simulink model "DynamicCompressionModel"  (R2019a)
settings: Solver=FixedStepDiscrete  StartTime=0.0  StopTime=t_end  RelTol=1e-3
InitFcn:
  | clear;
  | %DIAGNOSTIC = 0;  %% flag to give more information as simulation proceeds such as comments & plots
  | %CALIB_DIAGNOSTIC =  0; %% flag to give more information about calibration of filterbank due to overlap between filters: Mar 2016
  | %PRESCRIPT = 1;  %% flag to plot requested versus achieved insertion gains (esp for 125-250 Hz region).
  | %ipfiledigrms = -36; %% input file RMS in dB for 65 dB SPL equivalent
  | %opfiledigrms = -36; %% output file RMS in dB for 65 dB SPL equivalent
  | %equiv_ipSPL = 65; %% simulation of signal at this level through aid`
  | X_high = 1; % Maximum input
  | ref_dB = 85; X_ref = 1; % Define a reference point in X and its dBA value
  | % re_level = 10.^(.05*(equiv_ipSPL-65)); %% scale factor at start of hearing aid, to get input to desired simulation level
  | M_bits = 5;   % decides length of tables, 2^(4+M_bits)
  | 
  | NChans = 5;
  | [chan_cfs, ~ , t_atts, t_rels] ...
  |    = InitializeCompressionSettings(NChans);
  | % AidSettings5Chans;
  | 
  | %[VALID_WAV_FILE, sig, Fs, nbits, file_rms_dB, NStreams] ...
  | %  = loadwavfile(ipfiledigrms); %%  find [Fs], performs [recalculate] externally, provided valid file found
  | % VALID_WAV_FILE = 1;
  | [newfile, newpath] = uigetfile('*.wav','Open Signal File To Process.....');
  | if isequal(newfile,0) || isequal(newpath,0)
  |     fprintf(1,'\nFile not found'); VALID_WAV_FILE = 0;
  | else
  |     [sig, Fs] = audioread(strcat(newpath,newfile));
  | end
  | 
  | 
  | %% Test input: frequency sweep
  | X_thresh = 1*10^(0.05*(0-85));
  | Amplitudes = [X_thresh, X_thresh*10, X_thresh*100, X_thresh*1000, X_thresh*10000, 1]; %, X_thresh*100000];
  | 
  | %fMin = 100; %Hz
  | %fMax = 10000; %Hz
  | %Fs = 48000; %Hz
  | Fs_system = Fs;
  | Ts = 1/Fs;
  | Ts_system = Ts;
  | %tt = (0:length(sig)-1 )./Fs;
  | tt = 0:length(sig)-1;
  | tt = tt.*Ts;
  | %deltaF = (fMax - fMin)/tt(end);
  | %X_sweep = Amplitudes'*sin(2*pi*(fMin*tt +  0.5*deltaF*tt.*tt)) ;
  | 
  | %Volume = 6;
  | %sig = X_sweep(Volume,:)';
  | %% Replacing update_channel_params with only the needed pieces
  | 
  | % opplayer  = audioplayer(sig, Fs);
  | % nbits = opplayer.bitspersample;
  | %sig = resample(sig,48000,Fs);
  | %Fs = 48000;
  | 
  | 
  | % NStreams = min(size(sig));
  | EQ_SPAN_MSEC = 6;
  | 
  | insrt_frqs = [125, 250, 500, 1000, 2000, 3000, 4000, 6000, 8000, 10000 ]; %% decimal values
  | insrt_gns = [0 3 5 10 15 20 25 30 30 30]; %% prescribed dB for 65 dB input
  | %insrt_gns = 5*ones(1,length(insrt_frqs));  %no prescription
  | % n_insrts = length(insrt_gns);
  | 
  | UPPER_FREQ_LIM = min(11e3, 0.90*Fs/2);
  | 
  | % [ig_eq, calib_bpfs, dig_chan_lvl_0dBgain, dig_chan_dBthrs, Calib_recomb_dBpost] ...
  | %     = update_channel_params(Fs, NChans, chan_cfs, chan_thrs, insrt_frqs, insrt_gns, ...
  | %     0.1, UPPER_FREQ_LIM, EQ_SPAN_MSEC, PRESCRIPT, DIAGNOSTIC, CALIB_DIAGNOSTIC) ;  %% calculates channel edge frequencies, generates expected band levels for LTASS SWN to calibrate compressors & filterbank
  | [ig_eq, ~] = prescription_design_function(insrt_frqs, insrt_gns, Fs, EQ_SPAN_MSEC, 0); %% separate switch in [aid_sim] to turn off plotting.
  | %%% update_channel_params, to change edges array, as well as band levels when a channel cf changes.
  | edges = sqrt ( chan_cfs(2:end) .* chan_cfs(1:end-1) ); %% geometric mean
  | dummy_low_edge = edges(1)*(chan_cfs(1)/chan_cfs(2)); %% not used directly in Nchan_FbankAid, but helps with filter design, save for later
  | edges = [edges  UPPER_FREQ_LIM]; %% end stops to make software work, lowest not really implemented in software, upper set in main script
  | %%% spoof lowest edge freq for filyterbank design, not power calculations, does not produce edge in filterbank design
  | fb_edges = [dummy_low_edge  edges]; %% will need dummy low edge to make filterbank design software work, lowest not implemented in software other than transition width
  | [bpfs] = Nchan_FbankDesign(fb_edges, Fs, 0); %% Mar2016 move design of filterbank to here
  | 
  | calib_bpfs = bpfs; %% safety copy
  | % spec_size = 1024;
  | % bpzTotal= zeros(1,spec_size);
  | % bpCalzTotal = zeros(1,spec_size);
  | % Callibrate recombining gain? Or just fix bandpass FIRs to have unity peak gain.
  | % NOTE: Turns out bpfs have a pretty good peak unity gain. The combination
  | % of them all has a max error of -65 dBA (0.06%) above unity gain. That's fine.
  | %close(1); close(2);
  | % for(ix = 1:NChans)
  | %     [bpz(ix,:),bpFqs] = freqz(bpfs(2:(bpfs(1,ix)+1),ix),1,spec_size,Fs);
  | %     bpzMax(ix) = max(abs(bpz(ix,:)));
  | %     bpCalz(ix,:) = bpz(ix,:)./bpzMax(ix);
  | %     bpzTotal = bpzTotal + abs(bpz(ix,:));
  | %     bpCalzTotal = bpCalzTotal + abs(bpCalz(ix,:));
  | %     figure(1); hold on; semilogx(bpFqs, abs(bpz(ix,:)), 'b');
  | %     figure(2); hold on; semilogx(bpFqs, abs(bpCalz(ix,:)), 'g');
  | % end
  | % figure(1); hold on;
  | % semilogx(bpFqs, abs(bpzTotal), 'k'); %axis([100 12000 0 1.2]);
  | % xlabel('tested frqs(Hz)'); ylabel('Gain'); title('Original BP Response');
  | % figure(2); hold on;
  | % semilogx(bpFqs, abs(bpCalzTotal), 'k'); %axis([100 12000 0 1.2]);
  | % xlabel('tested frqs(Hz)'); ylabel('Gain'); title('Callibrated BP Response');
  | %%
  | 
  | % recombGain = 10.^(0.05.*Calib_recomb_dBpost);
  | recombGain = ones(1,NChans);
  | % translate sig into a form simulink likes
  | % Ts = 1/Fs;
  | % tt = (0:length(sig)-1).*Ts;
  | %t_end = tt(5*2^(M_bits+4) );   % to test table fill
  | t_end = tt(end);
  | sig_in = [tt', sig];
  | min_thresh_dB = 0;
  | for ix = 1:NChans
  |    [Gain_Table(:,ix), max_gain_prescript(ix), X_in(:,ix), chan_crs(ix)] ...
  |      = Compression_Wrapper_V2(Fs, min_thresh_dB, ...
  |      X_high, calib_bpfs(:,ix), ig_eq, ref_dB, X_ref, M_bits);
  | end
  | 
  | Initialize_Delay_Values;
  | %chan_recomb_gain = 10.^((0.05*Calib_recomb_dBpost));
  | W_bits = 32;
  | F_bits = 28;
  | M_bits = 5;
  | M_Bits = M_bits;
  | 
  | % Generating signals for simulink
  | Table_Fill = zeros(1,length(tt))';
  | %Table_Fill(1) = Gain_Table(end,5);
  | Table_Fill(1                : 2^(M_bits+4) )  = Gain_Table(:,1);
  | Table_Fill(2^(M_bits+4)+1   : 2*2^(M_bits+4) )= Gain_Table(:,2);
  | Table_Fill(2*2^(M_bits+4)+1 : 3*2^(M_bits+4) )= Gain_Table(:,3);
  | Table_Fill(3*2^(M_bits+4)+1 : 4*2^(M_bits+4) )= Gain_Table(:,4);
  | Table_Fill(4*2^(M_bits+4)+1 : 5*2^(M_bits+4) )= Gain_Table(:,5);
  | Table_Fill_t = [tt', zeros(1,length(tt))'];
  | Fill_Valid = zeros(1,length(tt))';
  | % Fill_Valid(1:5*2^(M_bits+4)) = 1;
  | % Fill_Valid = boolean(Fill_Valid);
  | Fill_Valid_t = [tt', Fill_Valid];
  | t_att = t_atts./1000; s_att = t_att.*Fs; % change units of t_atts from ms to samples
  | t_rel = t_rels./1000; s_rel = t_rel.*Fs; % change units of t_rels from ms to samples
  | r_att = nthroot(0.1, s_att);
  | r_rel = nthroot(0.1, s_rel);
  | 
  | Reset = [tt', boolean(zeros(1,length(tt)))'];
StopFcn:
  | proc_sig = double(out.proc_sig.data(:));
  | %alignedSigs = double(out.alignedSigs.data(:));
  | %[opwav, stop_ok] = savewavfile(opfiledigrms, ipfiledigrms, proc_sig, Fs, nbits, NStreams);
  | 
  | %load('SweepSimOutput.mat')
  | %X_out_Sweep_Sim(Volume,:) = proc_sig;
  | %save('SweepSimOutput.mat', 'X_out_Sweep_Sim');
values from neighbouring files (symbols this model uses):
  chan_cfs = [125 185 255 337 433 545 676 829 1008 1216 1460 1746 2079 2468 2923 3455 4077 4804 5653 6645 7805 9161]    [AidSettings22Chans.m]    (also in AidSettings3Chans.m = [750 1500 4000 ]; AidSettings5Chans.m = [500 1000 2000 4000 8000]; AidSettingsXChans.m = a*r.^(1:NChans); InitializeCompressionSettings.m = a*r.^(1:NChans))
  delayFix = maxDelay-delays    [Initialize_Delay_Values.m]    (also in cCompileTest.m = zeros(1,5))
  Fs = 48000    [cCompileTest.m]    (also in errorTesting.m; fft_compute_ASDF.m = 16000; fixedPointTesting.m; plotting_stuff.m)
  ig_eq = zeros(1,289)    [cCompileTest.m]
  sig = sig * 10.^(.05*adjustdB)    [loadwavfile.m]    (also in testing.m = X_sweep(Volume,:)')
  t_atts = [10 10 10 10 10 10 10 10 10 10 10 10 10 10 10 10 10 10 10 10 10 10]    [AidSettings22Chans.m]    (also in AidSettings3Chans.m = [200 100 100]; AidSettings5Chans.m = [200 100 100 100 100]; InitializeCompressionSettings.m = zeros(1,5))
  t_rels = [100 100 100 100 100 100 100 100 100 100 100 100 100 100 100 100 100 100 100 100 100 100]    [AidSettings22Chans.m]    (also in AidSettings3Chans.m = [2000 1500 1200 ]; AidSettings5Chans.m = [2000 1500 1200 1000 1000]; InitializeCompressionSettings.m = zeros(1,5))
libraries: simulink x352, hdlsllib x258, dsphdlfiltering x1
(part 1 of 7)
settings Model: DataTypeOverride=Off  Creator=Bailey  LastModifiedBy=Bailey
settings DataIOCC: InitialState=Table_Fill(1: 2^(M_bits+4) )  SaveOutput=off  SaveTime=off
settings OptimizationCC: BlockReduction=off  ConditionallyExecuteInputs=off  DefaultParameterBehavior=Inlined
settings DebuggingCC: AlgebraicLoopMsg=error  SingleTaskRateTransMsg=error
settings HardwareCC: ProdBitPerPointer=32  ProdBitPerSizeT=32  ProdBitPerPtrDiffT=32  ProdLargestAtomicFloat=None  ProdIntDivRoundTo=Undefined  ProdEndianess=Unspecified  ProdWordSize=32  ProdHWDeviceType=ASIC/FPGA->ASIC/FPGA  TargetBitPerPointer=64  TargetBitPerSizeT=64  TargetBitPerPtrDiffT=64  TargetLongLongMode=on  TargetIntDivRoundTo=Zero  TargetEndianess=LittleEndian  TargetWordSize=64  TargetHWDeviceType=Custom Processor->MATLAB Host Computer  ProdEqTarget=off

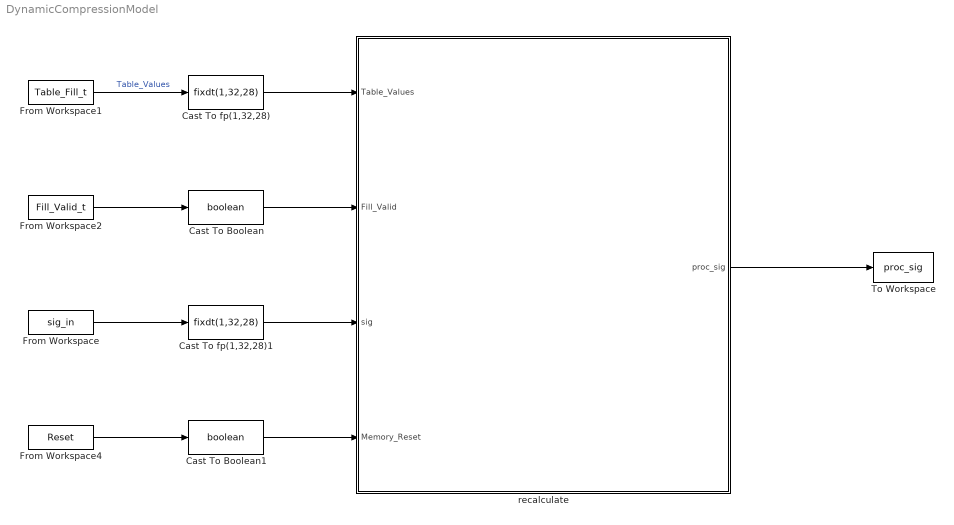
== system DynamicCompressionModel ==
  Cast To Boolean : DataTypeConversion  OutDataTypeStr=boolean
  Cast To Boolean1 : DataTypeConversion  OutDataTypeStr=boolean
  Cast To fp(1,32,28) : DataTypeConversion  OutDataTypeStr=fixdt(1,32,28)  RndMeth=Round
  Cast To fp(1,32,28)1 : DataTypeConversion  OutDataTypeStr=fixdt(1,32,28)  RndMeth=Round
  From Workspace : FromWorkspace  VariableName=sig_in  SampleTime=Ts  OutputAfterFinalValue=Setting to zero
  From Workspace1 : FromWorkspace  VariableName=Table_Fill_t  SampleTime=Ts  Interpolate=off  OutputAfterFinalValue=Setting to zero
  From Workspace2 : FromWorkspace  VariableName=Fill_Valid_t  SampleTime=Ts  OutputAfterFinalValue=Setting to zero
  From Workspace4 : FromWorkspace  VariableName=Reset  SampleTime=Ts  Interpolate=off  OutputAfterFinalValue=Setting to zero
  To Workspace : ToWorkspace  VariableName=proc_sig  SaveFormat=Timeseries  SampleTime=-1
  recalculate : Subsystem
  wires:
  From Workspace/1 -> Cast To fp(1,32,28)1/1
  recalculate/1(proc_sig) -> To Workspace/1
  From Workspace1/1 -> Cast To fp(1,32,28)/1  "Table_Values"
  From Workspace4/1 -> Cast To Boolean1/1
  Cast To Boolean/1 -> recalculate/2(Fill_Valid)
  From Workspace2/1 -> Cast To Boolean/1
  Cast To Boolean1/1 -> recalculate/4(Memory_Reset)
  Cast To fp(1,32,28)/1 -> recalculate/1(Table_Values)
  Cast To fp(1,32,28)1/1 -> recalculate/3(sig)

== system DynamicCompressionModel/recalculate ==
  note: High Clipping
  note: Prescription Application
  note: Low Clipping
  Table_Values : Inport
  Fill_Valid : Inport  Port=2
  sig : Inport  Port=3
  Memory_Reset : Inport  Port=4
  Compare To Constant : simulink/Logic and Bit Operations/Compare To Constant  relop=>=  const=X_high  OutDataTypeStr=boolean
  Compare To Constant1 : simulink/Logic and Bit Operations/Compare To Constant  relop=<=  const=-X_high  OutDataTypeStr=boolean
  Constant : Constant  Value=X_high  OutDataTypeStr=fixdt(1,W_bits, F_bits)  SampleTime=-1
  Constant1 : Constant  Value=-X_high  OutDataTypeStr=fixdt(1,W_bits, F_bits)  SampleTime=-1
  Nchan_FbankAGC_AID : Subsystem
  Switch : Switch  Criteria=u2 ~= 0
  Switch1 : Switch  Criteria=u2 ~= 0
  ig65 fir : DiscreteFir  Coefficients=ig_eq  CoefDataTypeStr=fixdt(1, W_bits*2, W_bits)  ProductDataTypeStr=fixdt(1, W_bits*2, W_bits)  AccumDataTypeStr=fixdt(1, W_bits*2, W_bits)  OutDataTypeStr=fixdt(1, W_bits, F_bits)
  proc_sig : Outport
  wires:
  sig/1 -> Nchan_FbankAGC_AID/3(input_signal)
  Table_Values/1 -> Nchan_FbankAGC_AID/1(Table_Values)
  Fill_Valid/1 -> Nchan_FbankAGC_AID/2(Fill_Valid)
  Memory_Reset/1 -> Nchan_FbankAGC_AID/4(Reset)
  ig65 fir/1 -> Compare To Constant/1, Switch/3  "re_level.*eq_sig"
  Nchan_FbankAGC_AID/1(proc_sig) -> ig65 fir/1
  Compare To Constant/1 -> Switch/2
  Constant/1 -> Switch/1
  Switch/1 -> Switch1/3, Compare To Constant1/1
  Compare To Constant1/1 -> Switch1/2
  Constant1/1 -> Switch1/1
  Switch1/1 -> proc_sig/1

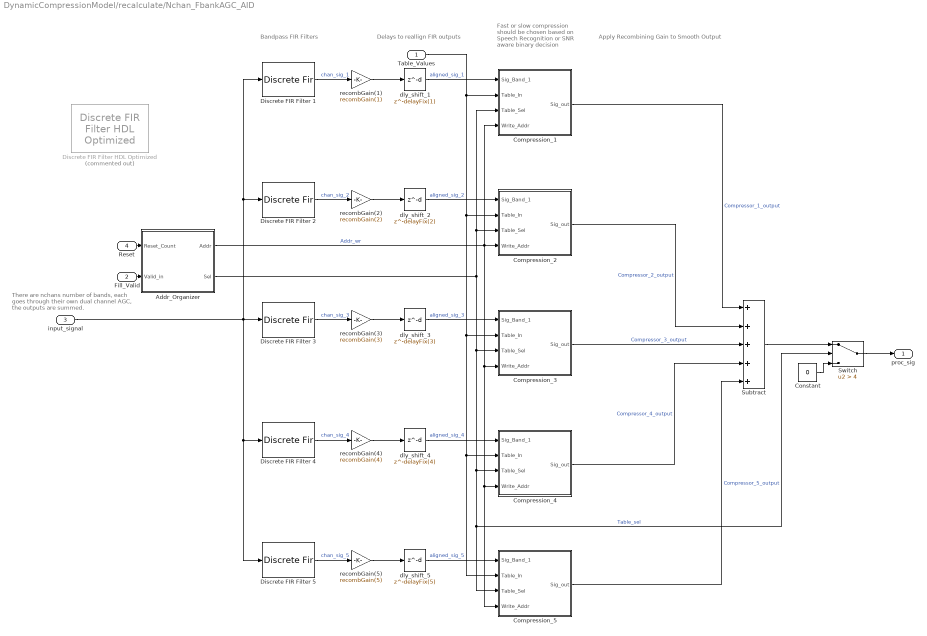
== system DynamicCompressionModel/recalculate/Nchan_FbankAGC_AID ==
  note: Apply Recombining Gain to Smooth Output
  note: Fast or slow compression
      | should be chosen based
      | on Speech Recognition or
      | SNR aware binary decision
  note: Delays to reallign FIR outputs
  note: Bandpass FIR Filters
  note: There are nchans number of bands,
      |  each goes through their own dual
      | channel AGC, the outputs are summed.
  Table_Values : Inport
  Fill_Valid : Inport  Port=2
  input_signal : Inport  Port=3
  Reset : Inport  Port=4
  Addr_Organizer : Subsystem
  Compression_1 : Subsystem
  Compression_2 : Subsystem
  Compression_3 : Subsystem
  Compression_4 : Subsystem
  Compression_5 : Subsystem
  Constant : Constant  Value=0  OutDataTypeStr=fixdt(1,W_bits, F_bits)  SampleTime=-1
  Discrete FIR Filter HDL Optimized : dsphdlfiltering/Discrete FIR Filter HDL Optimized  Commented=on  NumeratorSource=Property  Numerator=[ 0.5, 0.5 ]  NumeratorPrototype=[ 0.5, 0.5 ]  FilterStructure=Direct form systolic  SerializationOption=Minimum number of cycles between valid input samples  NumberOfCycles=2  NumberOfMultipliers=2  SimulateUsing=Code generation  roundingMode=Floor  overflowMode=off  CoefficientsDataTypeStr=Inherit: Same word length as input  CoefficientsMin=[]  CoefficientsMax=[]  OutputMin=[]  OutputMax=[]  ResetInputPort=off  HDLGlobalReset=off
      settings: SourceProductName=DSP System Toolbox  SourceProductBaseCode=DS
  Discrete FIR Filter 1 : DiscreteFir  Coefficients=calib_bpfs(2:calib_bpfs(1,1)+1 ,1)'  SampleTime=Ts  CoefDataTypeStr=fixdt(1, W_bits, F_bits)  ProductDataTypeStr=fixdt(1, W_bits, F_bits)  AccumDataTypeStr=fixdt(1, W_bits, F_bits)  OutDataTypeStr=fixdt(1, W_bits, F_bits)
  Discrete FIR Filter 2 : DiscreteFir  Coefficients=calib_bpfs(2:calib_bpfs(1,2)+1 ,2)'  CoefDataTypeStr=fixdt(1, W_bits, F_bits)  ProductDataTypeStr=fixdt(1, W_bits, F_bits)  AccumDataTypeStr=fixdt(1, W_bits, F_bits)  OutDataTypeStr=fixdt(1, W_bits, F_bits)
  Discrete FIR Filter 3 : DiscreteFir  Coefficients=calib_bpfs(2:calib_bpfs(1,3)+1 ,3)'  CoefDataTypeStr=fixdt(1, W_bits, F_bits)  ProductDataTypeStr=fixdt(1, W_bits, F_bits)  AccumDataTypeStr=fixdt(1, W_bits, F_bits)  OutDataTypeStr=fixdt(1, W_bits, F_bits)
  Discrete FIR Filter 4 : DiscreteFir  Coefficients=calib_bpfs(2:calib_bpfs(1,4)+1 ,4)'  CoefDataTypeStr=fixdt(1, W_bits, F_bits)  ProductDataTypeStr=fixdt(1, W_bits, F_bits)  AccumDataTypeStr=fixdt(1, W_bits, F_bits)  OutDataTypeStr=fixdt(1, W_bits, F_bits)
  Discrete FIR Filter 5 : DiscreteFir  Coefficients=calib_bpfs(2:calib_bpfs(1,5)+1 ,5)'  CoefDataTypeStr=fixdt(1, W_bits, F_bits)  ProductDataTypeStr=fixdt(1, W_bits, F_bits)  AccumDataTypeStr=fixdt(1, W_bits, F_bits)  OutDataTypeStr=fixdt(1, W_bits, F_bits)
  Subtract : Sum  Inputs=+++++
  Switch : Switch  Criteria=u2 > Threshold  Threshold=4
  dly_shift_1 : Delay  DelayLength=delayFix(1)  DelayLengthUpperLimit=500
  dly_shift_2 : Delay  DelayLength=delayFix(2)  DelayLengthUpperLimit=500
  dly_shift_3 : Delay  DelayLength=delayFix(3)  DelayLengthUpperLimit=500
  dly_shift_4 : Delay  DelayLength=delayFix(4)  DelayLengthUpperLimit=500
  dly_shift_5 : Delay  DelayLength=delayFix(5)  DelayLengthUpperLimit=500
  recombGain(1) : Gain  Gain=recombGain(1)  OutDataTypeStr=Inherit: Same as input
  recombGain(2) : Gain  Gain=recombGain(2)  OutDataTypeStr=Inherit: Same as input
  recombGain(3) : Gain  Gain=recombGain(3)  OutDataTypeStr=Inherit: Same as input
  recombGain(4) : Gain  Gain=recombGain(4)  OutDataTypeStr=Inherit: Same as input
  recombGain(5) : Gain  Gain=recombGain(5)  OutDataTypeStr=Inherit: Same as input
  proc_sig : Outport
  wires:
  Discrete FIR Filter 1/1 -> recombGain(1)/1  "chan_sig_1"
  dly_shift_1/1 -> Compression_1/1(Sig_Band_1)  "aligned_sig_1"
  Compression_1/1(Sig_out) -> Subtract/1  "Compressor_1_output"
  dly_shift_2/1 -> Compression_2/1(Sig_Band_1)  "aligned_sig_2"
  Discrete FIR Filter 2/1 -> recombGain(2)/1  "chan_sig_2"
  dly_shift_3/1 -> Compression_3/1(Sig_Band_1)  "aligned_sig_3"
  Discrete FIR Filter 3/1 -> recombGain(3)/1  "chan_sig_3"
  Discrete FIR Filter 5/1 -> recombGain(5)/1  "chan_sig_5"
  input_signal/1 -> Discrete FIR Filter 5/1, Discrete FIR Filter 4/1, Discrete FIR Filter 2/1, Discrete FIR Filter 1/1, Discrete FIR Filter 3/1
  dly_shift_5/1 -> Compression_5/1(Sig_Band_1)  "aligned_sig_5"
  dly_shift_4/1 -> Compression_4/1(Sig_Band_1)  "aligned_sig_4"
  Discrete FIR Filter 4/1 -> recombGain(4)/1  "chan_sig_4"
  Compression_3/1(Sig_out) -> Subtract/3  "Compressor_3_output"
  Compression_2/1(Sig_out) -> Subtract/2  "Compressor_2_output"
  Compression_4/1(Sig_out) -> Subtract/4  "Compressor_4_output"
  Compression_5/1(Sig_out) -> Subtract/5  "Compressor_5_output"
  Addr_Organizer/1(Addr) -> Compression_3/4(Write_Addr), Compression_5/4(Write_Addr), Compression_4/4(Write_Addr), Compression_2/4(Write_Addr), Compression_1/4(Write_Addr)  "Addr_wr"
  Reset/1 -> Addr_Organizer/1(Reset_Count)
  Fill_Valid/1 -> Addr_Organizer/2(Valid_in)
  Table_Values/1 -> Compression_5/2(Table_In), Compression_4/2(Table_In), Compression_3/2(Table_In), Compression_2/2(Table_In), Compression_1/2(Table_In)
  Addr_Organizer/2(Sel) -> Compression_3/3(Table_Sel), Compression_5/3(Table_Sel), Switch/2, Compression_4/3(Table_Sel), Compression_1/3(Table_Sel), Compression_2/3(Table_Sel)  "Table_sel"
  Subtract/1 -> Switch/1
  Constant/1 -> Switch/3
  Switch/1 -> proc_sig/1
  recombGain(1)/1 -> dly_shift_1/1
  recombGain(2)/1 -> dly_shift_2/1
  recombGain(3)/1 -> dly_shift_3/1
  recombGain(4)/1 -> dly_shift_4/1
  recombGain(5)/1 -> dly_shift_5/1

== system DynamicCompressionModel/recalculate/Nchan_FbankAGC_AID/Addr_Organizer ==
  note: Addr line contains the local address bits: 0-63
  note: Select Line is 000 to 101, if 110 writing is complete
  Reset_Count : Inport
  Valid_in : Inport  Port=2
  Bit Slice : hdlsllib/Logic and Bit Operations/Bit Slice  lidx=3+M_bits  ridx=0
      settings: SourceProductName=Simulink  SourceProductBaseCode=SL
  Bit Slice1 : hdlsllib/Logic and Bit Operations/Bit Slice  lidx=6+M_bits  ridx=4+M_bits
      settings: SourceProductName=Simulink  SourceProductBaseCode=SL
  Counter_up_to_320 : hdlsllib/Sources/HDL Counter  CountType=Count limited  CountInit=5*2^(4+M_Bits)  CountStep=1  CountMax=5*2^(4+M_Bits)+1  CountFromType=Initial value  CountFrom=5*2^(4+M_Bits)  CountResetPort=on  CountLoadPort=off  CountEnbPort=on  CountDirPort=off  CountDataType=Unsigned  CountWordLen=7+M_Bits  CountFracLen=0  CountSampTime=1
      settings: SourceProductName=Simulink
  Data Type Conversion : DataTypeConversion  OutDataTypeStr=fixdt(0,7+M_Bits,0)
  Data Type Conversion1 : DataTypeConversion  OutDataTypeStr=fixdt(0,4+M_bits,0)
  Data Type Conversion2 : DataTypeConversion  OutDataTypeStr=fixdt(0,3,0)
  Addr : Outport
  Sel : Outport  Port=2
  wires:
  Valid_in/1 -> Counter_up_to_320/2
  Reset_Count/1 -> Counter_up_to_320/1
  Counter_up_to_320/1 -> Data Type Conversion/1
  Data Type Conversion/1 -> Bit Slice1/1, Bit Slice/1
  Bit Slice1/1 -> Data Type Conversion2/1  "top3Bits"
  Bit Slice/1 -> Data Type Conversion1/1
  Data Type Conversion1/1 -> Addr/1
  Data Type Conversion2/1 -> Sel/1

== system DynamicCompressionModel/recalculate/Nchan_FbankAGC_AID/Compression_1 ==
  note: Calculate Compression Gain Needed
  note: Apply to the Envelope
  Sig_Band_1 : Inport
  Table_In : Inport  Port=2
  Table_Sel : Inport  Port=3
  Write_Addr : Inport  Port=4
  Compare To Constant : simulink/Logic and Bit Operations/Compare To Constant  relop===  const=0  OutDataTypeStr=boolean
  Compression_Envelope : Subsystem
  Compression_Gain_Calc : Subsystem
  Constant : Constant  Value=0  OutDataTypeStr=fixdt(1,W_bits,F_bits)  SampleTime=-1
  Data Type Conversion1 : DataTypeConversion  OutDataTypeStr=fixdt(1,W_bits,F_bits)
  Delay : Delay  DelayLength=3
  Product : Product
  Switch : Switch  Criteria=u2 > Threshold  Threshold=4  ZeroCross=off
  Unit Delay : UnitDelay  InitialCondition=1  SampleTime=-1  HasFrameUpgradeWarning=on
  Sig_out : Outport
  wires:
  Compression_Envelope/1(Gain_Out) -> Product/1, Unit Delay/1
  Unit Delay/1 -> Compression_Envelope/2(Curr_Gain)
  Product/1 -> Data Type Conversion1/1
  Compare To Constant/1 -> Compression_Gain_Calc/3(Table_Fill_Valid)
  Write_Addr/1 -> Compression_Gain_Calc/2(Write_Addr)
  Table_In/1 -> Compression_Gain_Calc/1(Table_Fill)  "Table_Values"
  Switch/1 -> Delay/1
  Table_Sel/1 -> Compare To Constant/1, Switch/2
  Constant/1 -> Switch/3
  Sig_Band_1/1 -> Compression_Gain_Calc/4(Data_In), Switch/1
  Data Type Conversion1/1 -> Sig_out/1
  Delay/1 -> Product/2
  Compression_Gain_Calc/1(Gain_C_out) -> Compression_Envelope/1(Desired_Gain)

== system DynamicCompressionModel/recalculate/Nchan_FbankAGC_AID/Compression_2 ==
  note: Calculate Compression Gain Needed
  note: Apply to the Envelope
  Sig_Band_1 : Inport
  Table_In : Inport  Port=2
  Table_Sel : Inport  Port=3
  Write_Addr : Inport  Port=4
  Compare To Constant : simulink/Logic and Bit Operations/Compare To Constant  relop===  const=1  OutDataTypeStr=boolean
  Compression_Envelope : Subsystem
  Compression_Gain_Calc : Subsystem
  Constant : Constant  Value=0  OutDataTypeStr=fixdt(1,W_bits,F_bits)  SampleTime=-1
  Data Type Conversion1 : DataTypeConversion  OutDataTypeStr=fixdt(1,W_bits,F_bits)
  Delay : Delay  DelayLength=3
  Product : Product
  Switch : Switch  Criteria=u2 > Threshold  Threshold=4  ZeroCross=off
  Unit Delay : UnitDelay  InitialCondition=1  SampleTime=-1  HasFrameUpgradeWarning=on
  Sig_out : Outport
  wires:
  Compression_Envelope/1(Gain_Out) -> Product/1, Unit Delay/1
  Unit Delay/1 -> Compression_Envelope/2(Curr_Gain)
  Compare To Constant/1 -> Compression_Gain_Calc/3(Table_Fill_Valid)
  Write_Addr/1 -> Compression_Gain_Calc/2(Write_Addr)
  Table_In/1 -> Compression_Gain_Calc/1(Table_Fill)  "Table_Values"
  Table_Sel/1 -> Compare To Constant/1, Switch/2
  Constant/1 -> Switch/3
  Switch/1 -> Delay/1
  Sig_Band_1/1 -> Compression_Gain_Calc/4(Data_In), Switch/1
  Product/1 -> Data Type Conversion1/1
  Data Type Conversion1/1 -> Sig_out/1
  Delay/1 -> Product/2
  Compression_Gain_Calc/1(Gain_C_out) -> Compression_Envelope/1(Desired_Gain)

== system DynamicCompressionModel/recalculate/Nchan_FbankAGC_AID/Compression_3 ==
  note: Calculate Compression Gain Needed
  note: Apply to the Envelope
  Sig_Band_1 : Inport
  Table_In : Inport  Port=2
  Table_Sel : Inport  Port=3
  Write_Addr : Inport  Port=4
  Compare To Constant : simulink/Logic and Bit Operations/Compare To Constant  relop===  const=2  OutDataTypeStr=boolean
  Compression_Envelope : Subsystem
  Compression_Gain_Calc : Subsystem
  Constant : Constant  Value=0  OutDataTypeStr=fixdt(1,W_bits,F_bits)  SampleTime=-1
  Data Type Conversion1 : DataTypeConversion  OutDataTypeStr=fixdt(1,W_bits,F_bits)
  Delay : Delay  DelayLength=3
  Product : Product
  Switch : Switch  Criteria=u2 > Threshold  Threshold=4  ZeroCross=off
  Unit Delay : UnitDelay  InitialCondition=1  SampleTime=-1  HasFrameUpgradeWarning=on
  Sig_out : Outport
  wires:
  Compression_Envelope/1(Gain_Out) -> Product/1, Unit Delay/1
  Unit Delay/1 -> Compression_Envelope/2(Curr_Gain)
  Compare To Constant/1 -> Compression_Gain_Calc/3(Table_Fill_Valid)
  Write_Addr/1 -> Compression_Gain_Calc/2(Write_Addr)
  Table_In/1 -> Compression_Gain_Calc/1(Table_Fill)  "Table_Values"
  Switch/1 -> Delay/1
  Table_Sel/1 -> Compare To Constant/1, Switch/2
  Constant/1 -> Switch/3
  Sig_Band_1/1 -> Compression_Gain_Calc/4(Data_In), Switch/1
  Product/1 -> Data Type Conversion1/1
  Data Type Conversion1/1 -> Sig_out/1
  Delay/1 -> Product/2
  Compression_Gain_Calc/1(Gain_C_out) -> Compression_Envelope/1(Desired_Gain)

== system DynamicCompressionModel/recalculate/Nchan_FbankAGC_AID/Compression_4 ==
  note: Calculate Compression Gain Needed
  note: Apply to the Envelope
  Sig_Band_1 : Inport
  Table_In : Inport  Port=2
  Table_Sel : Inport  Port=3
  Write_Addr : Inport  Port=4
  Compare To Constant : simulink/Logic and Bit Operations/Compare To Constant  relop===  const=3  OutDataTypeStr=boolean
  Compression_Envelope : Subsystem
  Compression_Gain_Calc : Subsystem
  Constant : Constant  Value=0  OutDataTypeStr=fixdt(1,W_bits,F_bits)  SampleTime=-1
  Data Type Conversion1 : DataTypeConversion  OutDataTypeStr=fixdt(1,W_bits,F_bits)
  Delay : Delay  DelayLength=3
  Product : Product
  Switch : Switch  Criteria=u2 > Threshold  Threshold=4  ZeroCross=off
  Unit Delay : UnitDelay  InitialCondition=1  SampleTime=-1  HasFrameUpgradeWarning=on
  Sig_out : Outport
  wires:
  Compression_Envelope/1(Gain_Out) -> Product/1, Unit Delay/1
  Unit Delay/1 -> Compression_Envelope/2(Curr_Gain)
  Compare To Constant/1 -> Compression_Gain_Calc/3(Table_Fill_Valid)
  Compression_Gain_Calc/1(Gain_C_out) -> Compression_Envelope/1(Desired_Gain)
  Write_Addr/1 -> Compression_Gain_Calc/2(Write_Addr)
  Table_In/1 -> Compression_Gain_Calc/1(Table_Fill)  "Table_Values"
  Switch/1 -> Delay/1
  Table_Sel/1 -> Compare To Constant/1, Switch/2
  Constant/1 -> Switch/3
  Sig_Band_1/1 -> Compression_Gain_Calc/4(Data_In), Switch/1
  Product/1 -> Data Type Conversion1/1
  Data Type Conversion1/1 -> Sig_out/1
  Delay/1 -> Product/2

== system DynamicCompressionModel/recalculate/Nchan_FbankAGC_AID/Compression_5 ==
  note: Calculate Compression Gain Needed
  note: Apply to the Envelope
  Sig_Band_1 : Inport
  Table_In : Inport  Port=2
  Table_Sel : Inport  Port=3
  Write_Addr : Inport  Port=4
  Compare To Constant : simulink/Logic and Bit Operations/Compare To Constant  relop===  const=4  OutDataTypeStr=boolean
  Compression_Envelope : Subsystem
  Compression_Gain_Calc : Subsystem
  Constant : Constant  Value=0  OutDataTypeStr=fixdt(1,W_bits,F_bits)  SampleTime=-1
  Data Type Conversion1 : DataTypeConversion  OutDataTypeStr=fixdt(1,W_bits,F_bits)
  Delay : Delay  DelayLength=3
  Product : Product
  Switch : Switch  Criteria=u2 > Threshold  Threshold=4  ZeroCross=off
  Unit Delay : UnitDelay  InitialCondition=1  SampleTime=-1  HasFrameUpgradeWarning=on
  Sig_out : Outport
  wires:
  Compression_Envelope/1(Gain_Out) -> Product/1, Unit Delay/1
  Unit Delay/1 -> Compression_Envelope/2(Curr_Gain)
  Compare To Constant/1 -> Compression_Gain_Calc/3(Table_Fill_Valid)
  Compression_Gain_Calc/1(Gain_C_out) -> Compression_Envelope/1(Desired_Gain)
  Write_Addr/1 -> Compression_Gain_Calc/2(Write_Addr)
  Table_In/1 -> Compression_Gain_Calc/1(Table_Fill)  "Table_Values"
  Switch/1 -> Delay/1
  Table_Sel/1 -> Compare To Constant/1, Switch/2
  Constant/1 -> Switch/3
  Sig_Band_1/1 -> Compression_Gain_Calc/4(Data_In), Switch/1
  Product/1 -> Data Type Conversion1/1
  Data Type Conversion1/1 -> Sig_out/1
  Delay/1 -> Product/2

== system DynamicCompressionModel/recalculate/Nchan_FbankAGC_AID/Compression_1/Compression_Envelope ==
  note: Curr > Desired:
      | Attack
  note: Curr < Desired:
      | Release
  Desired_Gain : Inport
  Curr_Gain : Inport  Port=2
  Attack_Envelope : Subsystem  TreatAsAtomicUnit=on
  Compare To Zero : simulink/Logic and Bit Operations/Compare To Zero  relop=>=  OutDataTypeStr=boolean
  Logical Operator : Logic  Operator=NOT  AllPortsSameDT=off  OutDataTypeStr=boolean
  Release_Envelope : Subsystem  TreatAsAtomicUnit=on
  Subtract : Sum  Inputs=-+  AccumDataTypeStr=fixdt(1,W_bits,F_bits)  OutDataTypeStr=Inherit: Same as accumulator
  Switch : Switch
  Gain_Out : Outport
  wires:
  Desired_Gain/1 -> Attack_Envelope/2(Desired), Release_Envelope/2(Desired), Subtract/1
  Curr_Gain/1 -> Attack_Envelope/1(Curr), Subtract/2, Release_Envelope/1(Curr)
  Subtract/1 -> Switch/2, Compare To Zero/1
  Compare To Zero/1 -> Attack_Envelope/Enable, Logical Operator/1
  Logical Operator/1 -> Release_Envelope/Enable
  Switch/1 -> Gain_Out/1
  Attack_Envelope/1(Gain_out) -> Switch/1
  Release_Envelope/1(Gain_out) -> Switch/3

== system DynamicCompressionModel/recalculate/Nchan_FbankAGC_AID/Compression_1/Compression_Gain_Calc ==
  note: Data_In assumed before applied prescription FIR
  note: Compression: Assume the input is a single band coming from the system.
      |
      | Goals:
      | 	- Take in a single point
      | 	- compare the volume to a known hard cap for the data
      | 	- attenuate the signal if it's above a certain threshold
      | 		- the distance above the threshold should be cut in dB by a ratio R
      | 	- return the output point at the same sample rate received
  Table_Fill : Inport
  Write_Addr : Inport  Port=2
  Table_Fill_Valid : Inport  Port=3
  Data_In : Inport  Port=4
  Abs : Abs
  Constant : Constant  OutDataTypeStr=fixdt(0,9,0)  SampleTime=-1
  High_Gain_Table : Subsystem  AncestorBlock=hdlsllibUNLOCKED/HDL RAMs/Dual Port RAM  mask(Dual-port RAM){ram_size=4+M_Bits}
      mask prompts: ram_size "Address port width (2 to 29 bits)"
      mask help: This block simulates a dual-port RAM with two data output ports.
      mask init:
      | hdlblkmask_dpram;
      mask Help: helpview([docroot '/simulink/helptargets.map'],'HDL_dual_port_RAM');
  Linear_Approximation : Subsystem
  LogAddressing : Subsystem
  Low_Gain_Table : Subsystem  mask(Dual-port RAM){ram_size=4+M_Bits}
      mask prompts: ram_size "Address port width (2 to 29 bits)"
      mask help: This block simulates a dual-port RAM with two data output ports.
      mask init:
      | hdlblkmask_dpram;
      mask Help: helpview([docroot '/simulink/helptargets.map'],'HDL_dual_port_RAM');
  Subtract : Sum  OutDataTypeStr=Inherit: Same as first input
  Terminator : Terminator
  Terminator1 : Terminator
  Unit Delay1 : UnitDelay  InitialCondition=1  SampleTime=-1  HasFrameUpgradeWarning=on
  Unit Delay2 : UnitDelay  InitialCondition=1  SampleTime=-1  HasFrameUpgradeWarning=on
  Unit Delay3 : UnitDelay  InitialCondition=1  SampleTime=-1  HasFrameUpgradeWarning=on
  Gain_C_out : Outport
  wires:
  Table_Fill/1 -> High_Gain_Table/1(wr_din), Low_Gain_Table/1(wr_din)
  Table_Fill_Valid/1 -> High_Gain_Table/3(wr_en), Low_Gain_Table/3(wr_en)
  Write_Addr/1 -> High_Gain_Table/2(wr_addr), Low_Gain_Table/2(wr_addr)
  LogAddressing/1(addr_r) -> Low_Gain_Table/4(rd_addr), Unit Delay3/1, Subtract/1  "addr_low"
  Abs/1 -> Unit Delay2/1, LogAddressing/1(x_in)  "|X_in|"
  Data_In/1 -> Abs/1
  Constant/1 -> Subtract/2
  Subtract/1 -> High_Gain_Table/4(rd_addr)  "addr_high"
  Low_Gain_Table/1(wr_dout) -> Terminator/1
  High_Gain_Table/1(wr_dout) -> Terminator1/1
  High_Gain_Table/2(rd_dout) -> Linear_Approximation/1(G_high)  "G_high"
  Low_Gain_Table/2(rd_dout) -> Linear_Approximation/2(G_low)  "G_low"
  Linear_Approximation/1(G_Desired) -> Gain_C_out/1
  Unit Delay2/1 -> Unit Delay1/1
  Unit Delay1/1 -> Linear_Approximation/4(|X_in|)
  Unit Delay3/1 -> Linear_Approximation/3(addr_low)

== system DynamicCompressionModel/recalculate/Nchan_FbankAGC_AID/Compression_2/Compression_Envelope ==
  note: Curr > Desired:
      | Attack
  note: Curr < Desired:
      | Release
  Desired_Gain : Inport
  Curr_Gain : Inport  Port=2
  Attack_Envelope : Subsystem  TreatAsAtomicUnit=on
  Compare To Zero : simulink/Logic and Bit Operations/Compare To Zero  relop=>=  OutDataTypeStr=boolean
  Logical Operator : Logic  Operator=NOT  AllPortsSameDT=off  OutDataTypeStr=boolean
  Release_Envelope : Subsystem  TreatAsAtomicUnit=on
  Subtract : Sum  Inputs=-+  AccumDataTypeStr=fixdt(1,W_bits,F_bits)  OutDataTypeStr=Inherit: Same as accumulator
  Switch : Switch
  Gain_Out : Outport
  wires:
  Desired_Gain/1 -> Attack_Envelope/2(Desired), Release_Envelope/2(Desired), Subtract/1
  Curr_Gain/1 -> Attack_Envelope/1(Curr), Subtract/2, Release_Envelope/1(Curr)
  Subtract/1 -> Switch/2, Compare To Zero/1
  Compare To Zero/1 -> Attack_Envelope/Enable, Logical Operator/1
  Logical Operator/1 -> Release_Envelope/Enable
  Switch/1 -> Gain_Out/1
  Attack_Envelope/1(Gain_out) -> Switch/1
  Release_Envelope/1(Gain_out) -> Switch/3

== system DynamicCompressionModel/recalculate/Nchan_FbankAGC_AID/Compression_2/Compression_Gain_Calc ==
  note: Data_In assumed before applied prescription FIR
  note: Compression: Assume the input is a single band coming from the system.
      |
      | Goals:
      | 	- Take in a single point
      | 	- compare the volume to a known hard cap for the data
      | 	- attenuate the signal if it's above a certain threshold
      | 		- the distance above the threshold should be cut in dB by a ratio R
      | 	- return the output point at the same sample rate received
  Table_Fill : Inport
  Write_Addr : Inport  Port=2
  Table_Fill_Valid : Inport  Port=3
  Data_In : Inport  Port=4
  Abs : Abs
  Constant : Constant  OutDataTypeStr=fixdt(0,9,0)  SampleTime=-1
  High_Gain_Table : Subsystem  AncestorBlock=hdlsllibUNLOCKED/HDL RAMs/Dual Port RAM  mask(Dual-port RAM){ram_size=4+M_Bits}
      mask prompts: ram_size "Address port width (2 to 29 bits)"
      mask help: This block simulates a dual-port RAM with two data output ports.
      mask init:
      | hdlblkmask_dpram;
      mask Help: helpview([docroot '/simulink/helptargets.map'],'HDL_dual_port_RAM');
  Linear_Approximation : Subsystem
  LogAddressing : Subsystem
  Low_Gain_Table : Subsystem  AncestorBlock=hdlsllibUNLOCKED/HDL RAMs/Dual Port RAM  mask(Dual-port RAM){ram_size=4+M_Bits}
      mask prompts: ram_size "Address port width (2 to 29 bits)"
      mask help: This block simulates a dual-port RAM with two data output ports.
      mask init:
      | hdlblkmask_dpram;
      mask Help: helpview([docroot '/simulink/helptargets.map'],'HDL_dual_port_RAM');
  Subtract : Sum  OutDataTypeStr=Inherit: Same as first input
  Terminator : Terminator
  Terminator1 : Terminator
  Unit Delay1 : UnitDelay  InitialCondition=1  SampleTime=-1  HasFrameUpgradeWarning=on
  Unit Delay2 : UnitDelay  InitialCondition=1  SampleTime=-1  HasFrameUpgradeWarning=on
  Unit Delay3 : UnitDelay  InitialCondition=1  SampleTime=-1  HasFrameUpgradeWarning=on
  Gain_C_out : Outport
  wires:
  Table_Fill/1 -> High_Gain_Table/1(wr_din), Low_Gain_Table/1(wr_din)
  Table_Fill_Valid/1 -> High_Gain_Table/3(wr_en), Low_Gain_Table/3(wr_en)
  Write_Addr/1 -> High_Gain_Table/2(wr_addr), Low_Gain_Table/2(wr_addr)
  LogAddressing/1(addr_r) -> Low_Gain_Table/4(rd_addr), Unit Delay3/1, Subtract/1  "addr_low"
  Abs/1 -> Unit Delay2/1, LogAddressing/1(x_in)  "|X_in|"
  Data_In/1 -> Abs/1
  Constant/1 -> Subtract/2
  Subtract/1 -> High_Gain_Table/4(rd_addr)  "addr_high"
  Low_Gain_Table/1(wr_dout) -> Terminator/1
  High_Gain_Table/1(wr_dout) -> Terminator1/1
  High_Gain_Table/2(rd_dout) -> Linear_Approximation/1(G_high)  "G_high"
  Low_Gain_Table/2(rd_dout) -> Linear_Approximation/2(G_low)  "G_low"
  Linear_Approximation/1(G_Desired) -> Gain_C_out/1
  Unit Delay2/1 -> Unit Delay1/1
  Unit Delay1/1 -> Linear_Approximation/4(|X_in|)
  Unit Delay3/1 -> Linear_Approximation/3(addr_low)

== system DynamicCompressionModel/recalculate/Nchan_FbankAGC_AID/Compression_3/Compression_Envelope ==
  note: Curr > Desired:
      | Attack
  note: Curr < Desired:
      | Release
  Desired_Gain : Inport
  Curr_Gain : Inport  Port=2
  Attack_Envelope : Subsystem  TreatAsAtomicUnit=on
  Compare To Zero : simulink/Logic and Bit Operations/Compare To Zero  relop=>=  OutDataTypeStr=boolean
  Logical Operator : Logic  Operator=NOT  AllPortsSameDT=off  OutDataTypeStr=boolean
  Release_Envelope : Subsystem  TreatAsAtomicUnit=on
  Subtract : Sum  Inputs=-+  AccumDataTypeStr=fixdt(1,W_bits,F_bits)  OutDataTypeStr=Inherit: Same as accumulator
  Switch : Switch
  Gain_Out : Outport
  wires:
  Desired_Gain/1 -> Attack_Envelope/2(Desired), Release_Envelope/2(Desired), Subtract/1
  Curr_Gain/1 -> Attack_Envelope/1(Curr), Subtract/2, Release_Envelope/1(Curr)
  Subtract/1 -> Switch/2, Compare To Zero/1
  Compare To Zero/1 -> Attack_Envelope/Enable, Logical Operator/1
  Logical Operator/1 -> Release_Envelope/Enable
  Switch/1 -> Gain_Out/1
  Attack_Envelope/1(Gain_out) -> Switch/1
  Release_Envelope/1(Gain_out) -> Switch/3

== system DynamicCompressionModel/recalculate/Nchan_FbankAGC_AID/Compression_3/Compression_Gain_Calc ==
  note: Data_In assumed before applied prescription FIR
  note: Compression: Assume the input is a single band coming from the system.
      |
      | Goals:
      | 	- Take in a single point
      | 	- compare the volume to a known hard cap for the data
      | 	- attenuate the signal if it's above a certain threshold
      | 		- the distance above the threshold should be cut in dB by a ratio R
      | 	- return the output point at the same sample rate received
  Table_Fill : Inport
  Write_Addr : Inport  Port=2
  Table_Fill_Valid : Inport  Port=3
  Data_In : Inport  Port=4
  Abs : Abs
  Constant : Constant  OutDataTypeStr=fixdt(0,9,0)  SampleTime=-1
  High_Gain_Table : Subsystem  AncestorBlock=hdlsllibUNLOCKED/HDL RAMs/Dual Port RAM  mask(Dual-port RAM){ram_size=4+M_Bits}
      mask prompts: ram_size "Address port width (2 to 29 bits)"
      mask help: This block simulates a dual-port RAM with two data output ports.
      mask init:
      | hdlblkmask_dpram;
      mask Help: helpview([docroot '/simulink/helptargets.map'],'HDL_dual_port_RAM');
  Linear_Approximation : Subsystem
  LogAddressing : Subsystem
  Low_Gain_Table : Subsystem  AncestorBlock=hdlsllibUNLOCKED/HDL RAMs/Dual Port RAM  mask(Dual-port RAM){ram_size=4+M_Bits}
      mask prompts: ram_size "Address port width (2 to 29 bits)"
      mask help: This block simulates a dual-port RAM with two data output ports.
      mask init:
      | hdlblkmask_dpram;
      mask Help: helpview([docroot '/simulink/helptargets.map'],'HDL_dual_port_RAM');
  Subtract : Sum  OutDataTypeStr=Inherit: Same as first input
  Terminator : Terminator
  Terminator1 : Terminator
  Unit Delay1 : UnitDelay  InitialCondition=1  SampleTime=-1  HasFrameUpgradeWarning=on
  Unit Delay2 : UnitDelay  InitialCondition=1  SampleTime=-1  HasFrameUpgradeWarning=on
  Unit Delay3 : UnitDelay  InitialCondition=1  SampleTime=-1  HasFrameUpgradeWarning=on
  Gain_C_out : Outport
  wires:
  Table_Fill/1 -> High_Gain_Table/1(wr_din), Low_Gain_Table/1(wr_din)
  Table_Fill_Valid/1 -> High_Gain_Table/3(wr_en), Low_Gain_Table/3(wr_en)
  Write_Addr/1 -> High_Gain_Table/2(wr_addr), Low_Gain_Table/2(wr_addr)
  LogAddressing/1(addr_r) -> Low_Gain_Table/4(rd_addr), Unit Delay3/1, Subtract/1  "addr_low"
  Abs/1 -> Unit Delay2/1, LogAddressing/1(x_in)  "|X_in|"
  Data_In/1 -> Abs/1
  Constant/1 -> Subtract/2
  Subtract/1 -> High_Gain_Table/4(rd_addr)  "addr_high"
  Low_Gain_Table/1(wr_dout) -> Terminator/1
  High_Gain_Table/1(wr_dout) -> Terminator1/1
  High_Gain_Table/2(rd_dout) -> Linear_Approximation/1(G_high)  "G_high"
  Low_Gain_Table/2(rd_dout) -> Linear_Approximation/2(G_low)  "G_low"
  Linear_Approximation/1(G_Desired) -> Gain_C_out/1
  Unit Delay2/1 -> Unit Delay1/1
  Unit Delay1/1 -> Linear_Approximation/4(|X_in|)
  Unit Delay3/1 -> Linear_Approximation/3(addr_low)

== system DynamicCompressionModel/recalculate/Nchan_FbankAGC_AID/Compression_4/Compression_Envelope ==
  note: Curr > Desired:
      | Attack
  note: Curr < Desired:
      | Release
  Desired_Gain : Inport
  Curr_Gain : Inport  Port=2
  Attack_Envelope : Subsystem  TreatAsAtomicUnit=on
  Compare To Zero : simulink/Logic and Bit Operations/Compare To Zero  relop=>=  OutDataTypeStr=boolean
  Logical Operator : Logic  Operator=NOT  AllPortsSameDT=off  OutDataTypeStr=boolean
  Release_Envelope : Subsystem  TreatAsAtomicUnit=on
  Subtract : Sum  Inputs=-+  AccumDataTypeStr=fixdt(1,W_bits,F_bits)  OutDataTypeStr=Inherit: Same as accumulator
  Switch : Switch
  Gain_Out : Outport
  wires:
  Desired_Gain/1 -> Attack_Envelope/2(Desired), Release_Envelope/2(Desired), Subtract/1
  Curr_Gain/1 -> Attack_Envelope/1(Curr), Subtract/2, Release_Envelope/1(Curr)
  Subtract/1 -> Switch/2, Compare To Zero/1
  Compare To Zero/1 -> Attack_Envelope/Enable, Logical Operator/1
  Logical Operator/1 -> Release_Envelope/Enable
  Switch/1 -> Gain_Out/1
  Attack_Envelope/1(Gain_out) -> Switch/1
  Release_Envelope/1(Gain_out) -> Switch/3

== system DynamicCompressionModel/recalculate/Nchan_FbankAGC_AID/Compression_4/Compression_Gain_Calc ==
  note: Data_In assumed before applied prescription FIR
  note: Compression: Assume the input is a single band coming from the system.
      |
      | Goals:
      | 	- Take in a single point
      | 	- compare the volume to a known hard cap for the data
      | 	- attenuate the signal if it's above a certain threshold
      | 		- the distance above the threshold should be cut in dB by a ratio R
      | 	- return the output point at the same sample rate received
  Table_Fill : Inport
  Write_Addr : Inport  Port=2
  Table_Fill_Valid : Inport  Port=3
  Data_In : Inport  Port=4
  Abs : Abs
  Constant : Constant  OutDataTypeStr=fixdt(0,9,0)  SampleTime=-1
  High_Gain_Table : Subsystem  AncestorBlock=hdlsllibUNLOCKED/HDL RAMs/Dual Port RAM  mask(Dual-port RAM){ram_size=4+M_Bits}
      mask prompts: ram_size "Address port width (2 to 29 bits)"
      mask help: This block simulates a dual-port RAM with two data output ports.
      mask init:
      | hdlblkmask_dpram;
      mask Help: helpview([docroot '/simulink/helptargets.map'],'HDL_dual_port_RAM');
  Linear_Approximation : Subsystem
  LogAddressing : Subsystem
  Low_Gain_Table : Subsystem  AncestorBlock=hdlsllibUNLOCKED/HDL RAMs/Dual Port RAM  mask(Dual-port RAM){ram_size=4+M_Bits}
      mask prompts: ram_size "Address port width (2 to 29 bits)"
      mask help: This block simulates a dual-port RAM with two data output ports.
      mask init:
      | hdlblkmask_dpram;
      mask Help: helpview([docroot '/simulink/helptargets.map'],'HDL_dual_port_RAM');
  Subtract : Sum  OutDataTypeStr=Inherit: Same as first input
  Terminator : Terminator
  Terminator1 : Terminator
  Unit Delay1 : UnitDelay  InitialCondition=1  SampleTime=-1  HasFrameUpgradeWarning=on
  Unit Delay2 : UnitDelay  InitialCondition=1  SampleTime=-1  HasFrameUpgradeWarning=on
  Unit Delay3 : UnitDelay  InitialCondition=1  SampleTime=-1  HasFrameUpgradeWarning=on
  Gain_C_out : Outport
  wires:
  Table_Fill/1 -> High_Gain_Table/1(wr_din), Low_Gain_Table/1(wr_din)
  Table_Fill_Valid/1 -> High_Gain_Table/3(wr_en), Low_Gain_Table/3(wr_en)
  Write_Addr/1 -> High_Gain_Table/2(wr_addr), Low_Gain_Table/2(wr_addr)
  LogAddressing/1(addr_r) -> Low_Gain_Table/4(rd_addr), Unit Delay3/1, Subtract/1  "addr_low"
  Abs/1 -> Unit Delay2/1, LogAddressing/1(x_in)  "|X_in|"
  Data_In/1 -> Abs/1
  Constant/1 -> Subtract/2
  Subtract/1 -> High_Gain_Table/4(rd_addr)  "addr_high"
  Low_Gain_Table/1(wr_dout) -> Terminator/1
  High_Gain_Table/1(wr_dout) -> Terminator1/1
  High_Gain_Table/2(rd_dout) -> Linear_Approximation/1(G_high)  "G_high"
  Low_Gain_Table/2(rd_dout) -> Linear_Approximation/2(G_low)  "G_low"
  Linear_Approximation/1(G_Desired) -> Gain_C_out/1
  Unit Delay2/1 -> Unit Delay1/1
  Unit Delay1/1 -> Linear_Approximation/4(|X_in|)
  Unit Delay3/1 -> Linear_Approximation/3(addr_low)

== system DynamicCompressionModel/recalculate/Nchan_FbankAGC_AID/Compression_5/Compression_Envelope ==
  note: Curr > Desired:
      | Attack
  note: Curr < Desired:
      | Release
  Desired_Gain : Inport
  Curr_Gain : Inport  Port=2
  Attack_Envelope : Subsystem  TreatAsAtomicUnit=on
  Compare To Zero : simulink/Logic and Bit Operations/Compare To Zero  relop=>=  OutDataTypeStr=boolean
  Logical Operator : Logic  Operator=NOT  AllPortsSameDT=off  OutDataTypeStr=boolean
  Release_Envelope : Subsystem  TreatAsAtomicUnit=on
  Subtract : Sum  Inputs=-+  AccumDataTypeStr=fixdt(1,W_bits,F_bits)  OutDataTypeStr=Inherit: Same as accumulator
  Switch : Switch
  Gain_Out : Outport
  wires:
  Desired_Gain/1 -> Attack_Envelope/2(Desired), Release_Envelope/2(Desired), Subtract/1
  Curr_Gain/1 -> Attack_Envelope/1(Curr), Subtract/2, Release_Envelope/1(Curr)
  Subtract/1 -> Switch/2, Compare To Zero/1
  Compare To Zero/1 -> Attack_Envelope/Enable, Logical Operator/1
  Logical Operator/1 -> Release_Envelope/Enable
  Switch/1 -> Gain_Out/1
  Attack_Envelope/1(Gain_out) -> Switch/1
  Release_Envelope/1(Gain_out) -> Switch/3

== system DynamicCompressionModel/recalculate/Nchan_FbankAGC_AID/Compression_5/Compression_Gain_Calc ==
  note: Data_In assumed before applied prescription FIR
  note: Compression: Assume the input is a single band coming from the system.
      |
      | Goals:
      | 	- Take in a single point
      | 	- compare the volume to a known hard cap for the data
      | 	- attenuate the signal if it's above a certain threshold
      | 		- the distance above the threshold should be cut in dB by a ratio R
      | 	- return the output point at the same sample rate received
  Table_Fill : Inport
  Write_Addr : Inport  Port=2
  Table_Fill_Valid : Inport  Port=3
  Data_In : Inport  Port=4
  Abs : Abs
  Constant : Constant  OutDataTypeStr=fixdt(0,9,0)  SampleTime=-1
  High_Gain_Table : Subsystem  AncestorBlock=hdlsllibUNLOCKED/HDL RAMs/Dual Port RAM  mask(Dual-port RAM){ram_size=4+M_Bits}
      mask prompts: ram_size "Address port width (2 to 29 bits)"
      mask help: This block simulates a dual-port RAM with two data output ports.
      mask init:
      | hdlblkmask_dpram;
      mask Help: helpview([docroot '/simulink/helptargets.map'],'HDL_dual_port_RAM');
  Linear_Approximation : Subsystem
  LogAddressing : Subsystem
  Low_Gain_Table : Subsystem  AncestorBlock=hdlsllibUNLOCKED/HDL RAMs/Dual Port RAM  mask(Dual-port RAM){ram_size=4+M_Bits}
      mask prompts: ram_size "Address port width (2 to 29 bits)"
      mask help: This block simulates a dual-port RAM with two data output ports.
      mask init:
      | hdlblkmask_dpram;
      mask Help: helpview([docroot '/simulink/helptargets.map'],'HDL_dual_port_RAM');
  Subtract : Sum  OutDataTypeStr=Inherit: Same as first input
  Terminator : Terminator
  Terminator1 : Terminator
  Unit Delay1 : UnitDelay  InitialCondition=1  SampleTime=-1  HasFrameUpgradeWarning=on
  Unit Delay2 : UnitDelay  InitialCondition=1  SampleTime=-1  HasFrameUpgradeWarning=on
  Unit Delay3 : UnitDelay  InitialCondition=1  SampleTime=-1  HasFrameUpgradeWarning=on
  Gain_C_out : Outport
  wires:
  Table_Fill/1 -> High_Gain_Table/1(wr_din), Low_Gain_Table/1(wr_din)
  Table_Fill_Valid/1 -> High_Gain_Table/3(wr_en), Low_Gain_Table/3(wr_en)
  Write_Addr/1 -> High_Gain_Table/2(wr_addr), Low_Gain_Table/2(wr_addr)
  LogAddressing/1(addr_r) -> Low_Gain_Table/4(rd_addr), Unit Delay3/1, Subtract/1  "addr_low"
  Abs/1 -> Unit Delay2/1, LogAddressing/1(x_in)  "|X_in|"
  Data_In/1 -> Abs/1
  Constant/1 -> Subtract/2
  Subtract/1 -> High_Gain_Table/4(rd_addr)  "addr_high"
  Low_Gain_Table/1(wr_dout) -> Terminator/1
  High_Gain_Table/1(wr_dout) -> Terminator1/1
  High_Gain_Table/2(rd_dout) -> Linear_Approximation/1(G_high)  "G_high"
  Low_Gain_Table/2(rd_dout) -> Linear_Approximation/2(G_low)  "G_low"
  Linear_Approximation/1(G_Desired) -> Gain_C_out/1
  Unit Delay2/1 -> Unit Delay1/1
  Unit Delay1/1 -> Linear_Approximation/4(|X_in|)
  Unit Delay3/1 -> Linear_Approximation/3(addr_low)

== system DynamicCompressionModel/recalculate/Nchan_FbankAGC_AID/Compression_1/Compression_Envelope/Attack_Envelope ==
  note: ATTACK
  Curr : Inport
  Desired : Inport  Port=2
  Enable : EnablePort
  Product : Product  OutDataTypeStr=Inherit: Same as first input
  Subtract : Sum  Inputs=+-
  Subtract1 : Sum  OutDataTypeStr=fixdt(1,W_bits, F_bits)
  r_att(1) : Constant  Value=r_att(1)  OutDataTypeStr=fixdt(1,W_bits*2,W_bits+F_bits)  SampleTime=-1
  Gain_out : Outport  InitialOutput=0
  wires:
  Desired/1 -> Subtract/2, Subtract1/2
  Curr/1 -> Subtract/1
  Subtract/1 -> Product/2
  r_att(1)/1 -> Product/1
  Product/1 -> Subtract1/1  "Apply_Envelope"
  Subtract1/1 -> Gain_out/1

== system DynamicCompressionModel/recalculate/Nchan_FbankAGC_AID/Compression_1/Compression_Envelope/Release_Envelope ==
  note: RELEASE
  Curr : Inport
  Desired : Inport  Port=2
  Enable : EnablePort
  Product : Product  OutDataTypeStr=Inherit: Same as first input
  Subtract : Sum  Inputs=+-
  Subtract1 : Sum  Inputs=+-  OutDataTypeStr=Inherit: Same as first input
  r_rel(1) : Constant  Value=r_rel(1)  OutDataTypeStr=fixdt(1,W_bits*2,W_bits+F_bits)  SampleTime=-1
  Gain_out : Outport  InitialOutput=0
  wires:
  Desired/1 -> Subtract1/1, Subtract/1
  Curr/1 -> Subtract/2
  Subtract/1 -> Product/1
  r_rel(1)/1 -> Product/2
  Product/1 -> Subtract1/2  "Apply_Envelope"
  Subtract1/1 -> Gain_out/1
